simulink model "mask_test"  (R2022a)
settings: Solver=FixedStepDiscrete  StartTime=0.0  StopTime=10.0  RelTol=1e-3
PreLoadFcn:
  | mask_initialized = 0;
  | Local_test = 3;
InitFcn:
  | mask_initialized = 0;
  | Local_test = 3;
libraries: shared_library x3
settings Model: Creator=KenYoshioka  LastModifiedBy=KenYoshioka
settings OptimizationCC: DefaultParameterBehavior=Inlined  EnhancedBackFolding=on  PassReuseOutputArgsAs=Individual arguments  ZeroExternalMemoryAtStartup=off  ZeroInternalMemoryAtStartup=off  OptimizeBlockOrder=speed  DifferentSizesBufferReuse=on  OptimizationCustomize=off  EfficientTunableParamExpr=on
settings DebuggingCC: ParameterTunabilityLossMsg=error
settings SFSimCC: MATLABDynamicMemAlloc=off
settings RTWCC: SystemTargetFile=ert.tlc  TemplateMakefile=ert_default_tmf
settings CodeAppCC: ForceParamTrailComments=on  IgnoreCustomStorageClasses=off  OperatorAnnotations=on  SimulinkDataObjDesc=on  SFDataObjDesc=on  InsertBlockDesc=on
settings ERTTargetCC: TargetLangStandard=C99 (ISO)  GenerateSampleERTMain=on  InlinedParameterPlacement=NonHierarchical  ERTCustomFileTemplate=example_file_process.tlc

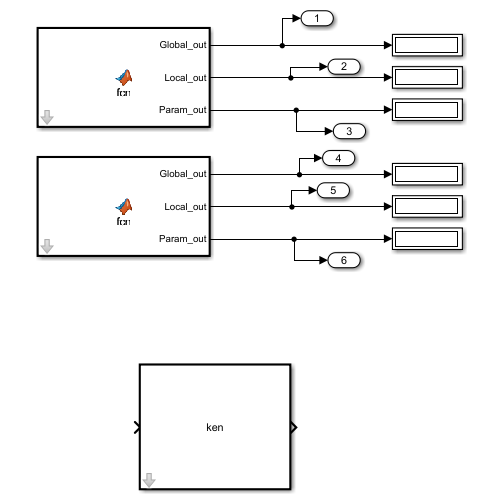
[thumbnail: Simulink's stored preview of the top-level diagram]
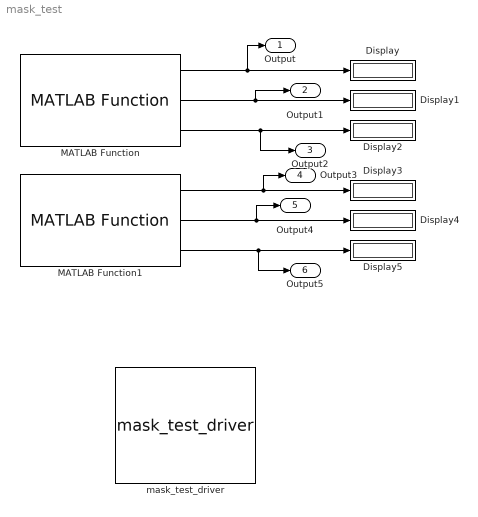
== system mask_test ==
  Display{,1..5} (6 alike) : Display
  MATLAB Function : shared_library/MATLAB Function  Param_test=0
  MATLAB Function1 : shared_library/MATLAB Function  Param_test=0
  mask_test_driver : shared_library/mask_test_driver  Param_init=2
  Output : Outport
  Output1 : Outport  Port=2
  Output2 : Outport  Port=3
  Output3 : Outport  Port=4
  Output4 : Outport  Port=5
  Output5 : Outport  Port=6
  wires:
  MATLAB Function/1 -> Output/1, Display/1
  MATLAB Function/2 -> Output1/1, Display1/1
  MATLAB Function/3 -> Output2/1, Display2/1
  MATLAB Function1/1 -> Output3/1, Display3/1
  MATLAB Function1/3 -> Output5/1, Display5/1
  MATLAB Function1/2 -> Output4/1, Display4/1
